simulink model "gm_DVBS_AXI4Stream"  (R2023b)
settings: Solver=FixedStepAuto  StartTime=0.0  StopTime=160000/fs  FixedStep=5e-9  RelTol=1e-3  EnableMultiTasking=on
model workspace (MAT data in the model file):
  HDLVAXIManagerConfig = hdlverifier.internal.AXIMaster.ConfigParams
undefined symbols (not defined in the file or in its folder): ctrlIn, fs, iniStates, n, sourceData
libraries: simulink x12, hdlsllib x9, whdledac x1, commcnvintrlv2 x1, commhdlblkcod x1
settings Model: Creator=31651  LastModifiedBy=31651
settings SolverCC: PositivePriorityOrder=on  AutoInsertRateTranBlk=on
settings DataIOCC: ReturnWorkspaceOutputs=off
settings OptimizationCC: BlockReduction=off  ConditionallyExecuteInputs=off  DefaultParameterBehavior=Inlined  DefaultUnderspecifiedDataType=single  EnhancedBackFolding=on  PassReuseOutputArgsAs=Individual arguments  ZeroExternalMemoryAtStartup=off  ZeroInternalMemoryAtStartup=off  MaxStackSize=64  OptimizeBlockOrder=speed  DifferentSizesBufferReuse=on  OptimizationCustomize=off  EfficientTunableParamExpr=on
settings DebuggingCC: AlgebraicLoopMsg=error  ArtificialAlgebraicLoopMsg=none  InheritedTsInSrcMsg=none  SingleTaskRateTransMsg=error  ParameterPrecisionLossMsg=none  ParameterTunabilityLossMsg=error
settings HardwareCC: ProdBitPerPointer=32  ProdBitPerSizeT=32  ProdBitPerPtrDiffT=32  ProdLargestAtomicFloat=None  ProdIntDivRoundTo=Undefined  ProdEndianess=Unspecified  ProdWordSize=32  ProdHWDeviceType=ASIC/FPGA->ASIC/FPGA  TargetBitPerPointer=64  TargetBitPerSizeT=64  TargetBitPerPtrDiffT=64  TargetLongLongMode=on  TargetIntDivRoundTo=Zero  TargetEndianess=LittleEndian  TargetWordSize=64  TargetHWDeviceType=Custom Processor->MATLAB Host Computer  ProdEqTarget=off  HardwareBoardFeatureSet=SoCBlockset
settings ModelReferenceCC: ModelReferenceNumInstancesAllowed=Single
settings SFSimCC: MATLABDynamicMemAlloc=off
settings RTWCC: Description=Embedded Coder  SystemTargetFile=ert.tlc  TemplateMakefile=ert_default_tmf
settings CodeAppCC: ForceParamTrailComments=on  IgnoreCustomStorageClasses=off  OperatorAnnotations=on  SimulinkDataObjDesc=on  SFDataObjDesc=on  InsertBlockDesc=on
settings ERTTargetCC: ERTCustomFileTemplate=example_file_process.tlc

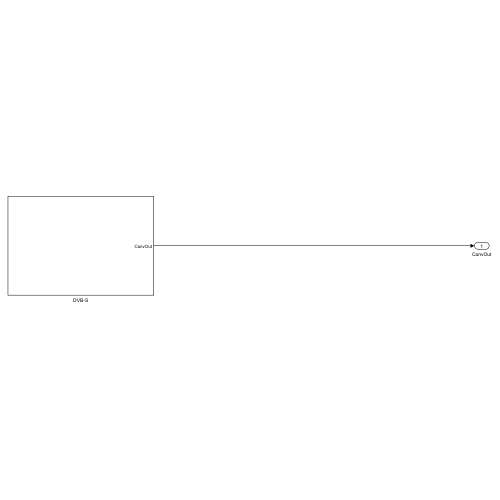
[thumbnail: Simulink's stored preview of the top-level diagram]
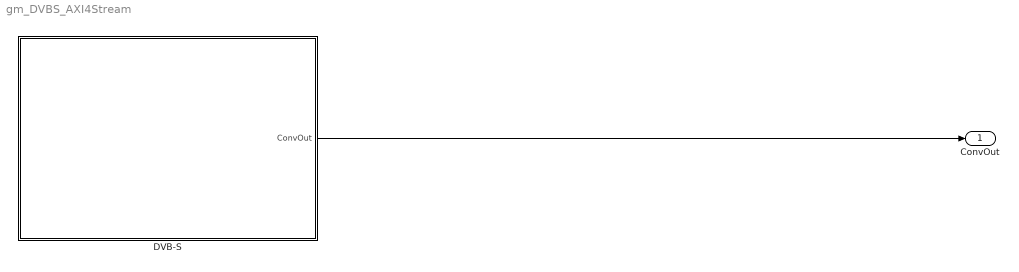
== system gm_DVBS_AXI4Stream ==
  DVB-S : Subsystem
  ConvOut : Outport  VectorParamsAs1DForOutWhenUnconnected=off
  wires:
  DVB-S/1(ConvOut) -> ConvOut/1

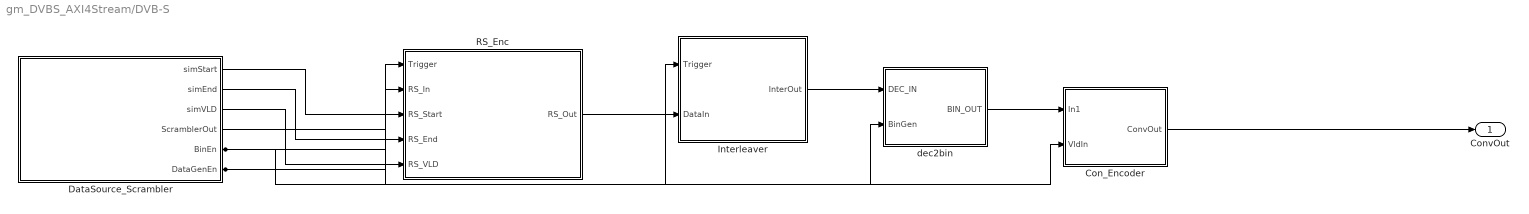
== system gm_DVBS_AXI4Stream/DVB-S ==
  Con_Encoder : Subsystem
  DataSource_Scrambler : Subsystem
  Interleaver : Subsystem
  RS_Enc : Subsystem
  dec2bin : Subsystem
  ConvOut : Outport  SampleTime=5e-09
  wires:
  Con_Encoder/1(ConvOut) -> ConvOut/1
  DataSource_Scrambler/1(simStart) -> RS_Enc/3(RS_Start)
  DataSource_Scrambler/2(simEnd) -> RS_Enc/4(RS_End)
  DataSource_Scrambler/3("simVLD ") -> RS_Enc/5(RS_VLD)
  DataSource_Scrambler/4(ScramblerOut) -> RS_Enc/2(RS_In)
  DataSource_Scrambler/5(BinEn) -> Con_Encoder/2(VldIn), dec2bin/2(BinGen)
  DataSource_Scrambler/6(DataGenEn) -> RS_Enc/1(Trigger), Interleaver/1(Trigger)
  Interleaver/1(InterOut) -> dec2bin/1(DEC_IN)
  RS_Enc/1(RS_Out) -> Interleaver/2(DataIn)
  dec2bin/1(BIN_OUT) -> Con_Encoder/1(In1)

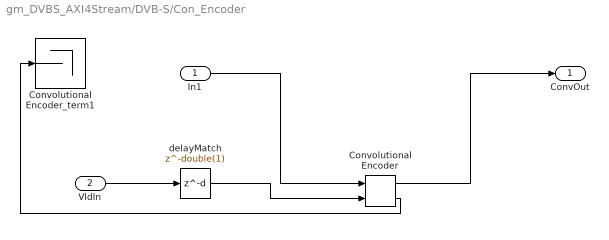
== system gm_DVBS_AXI4Stream/DVB-S/Con_Encoder ==
  In1 : Inport  OutDataTypeStr=boolean  PortDimensions=1  SampleTime=5e-09
  VldIn : Inport  Port=2  OutDataTypeStr=boolean  PortDimensions=1  SampleTime=5e-09
  Convolutional Encoder : whdledac/Convolutional Encoder  ConstraintLength=7  CodeGenerator=[171 133]  FeedbackConnection=0  TerminationMethod=Continuous  ResetPort=off  InitialStatePort=off  FinalStatePort=off  SimulateUsing=Code generation
  Convolutional Encoder_term1 : Terminator
  delayMatch : Delay  DelayLength=double(1)  InitialCondition=0  SampleTime=5e-09
  ConvOut : Outport  SampleTime=5e-09
  wires:
  In1/1 -> Convolutional Encoder/1
  delayMatch/1 -> Convolutional Encoder/2
  Convolutional Encoder/1 -> ConvOut/1
  Convolutional Encoder/2 -> Convolutional Encoder_term1/1
  VldIn/1 -> delayMatch/1

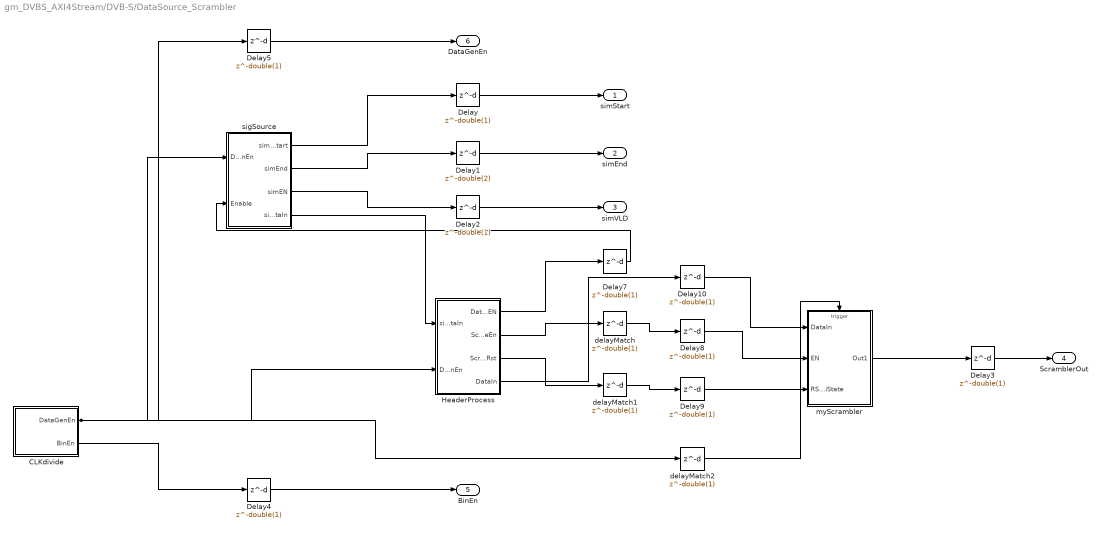
== system gm_DVBS_AXI4Stream/DVB-S/DataSource_Scrambler ==
  CLKdivide : Subsystem
  Delay{,2..5,7..10} (9 alike) : Delay  DelayLength=double(1)  InitialCondition=0  SampleTime=5e-09
  Delay1 : Delay  DelayLength=double(2)  InitialCondition=0  SampleTime=5e-09
  HeaderProcess : Subsystem
  delayMatch : Delay  DelayLength=double(1)  InitialCondition=0  SampleTime=5e-09
  delayMatch1 : Delay  DelayLength=double(1)  InitialCondition=0  SampleTime=5e-09
  delayMatch2 : Delay  DelayLength=double(1)  InitialCondition=0  SampleTime=5e-09
  myScrambler : Subsystem
  sigSource : Subsystem
  simStart : Outport  SampleTime=5e-09
  simEnd : Outport  Port=2  SampleTime=5e-09
  "simVLD " : Outport  Port=3  SampleTime=5e-09
  ScramblerOut : Outport  Port=4  SampleTime=5e-09
  BinEn : Outport  Port=5  SampleTime=5e-09  VectorParamsAs1DForOutWhenUnconnected=off
  DataGenEn : Outport  Port=6  SampleTime=5e-09  VectorParamsAs1DForOutWhenUnconnected=off
  wires:
  delayMatch2/1 -> myScrambler/Trigger
  CLKdivide/2(BinEn) -> Delay4/1
  Delay/1 -> simStart/1
  Delay1/1 -> simEnd/1
  Delay10/1 -> myScrambler/1(DataIn)
  Delay2/1 -> "simVLD "/1
  Delay3/1 -> ScramblerOut/1
  Delay4/1 -> BinEn/1
  Delay5/1 -> DataGenEn/1
  Delay8/1 -> myScrambler/2(EN)
  Delay9/1 -> myScrambler/3(RST_IniState)
  myScrambler/1(Out1) -> Delay3/1
  CLKdivide/1(DataGenEn) -> delayMatch2/1, Delay5/1, sigSource/1(DataGenEn), HeaderProcess/2(DataGenEn)
  delayMatch/1 -> Delay8/1
  delayMatch1/1 -> Delay9/1
  HeaderProcess/1(DataGenEN) -> Delay7/1
  sigSource/1(simStart) -> Delay/1
  sigSource/2(simEnd) -> Delay1/1
  sigSource/3(simEN) -> Delay2/1
  Delay7/1 -> sigSource/2(Enable)
  HeaderProcess/2(ScrambleEn) -> delayMatch/1
  HeaderProcess/3(ScrambleRst) -> delayMatch1/1
  HeaderProcess/4(DataIn) -> Delay10/1
  sigSource/4(simDataIn) -> HeaderProcess/1(simDataIn)

== system gm_DVBS_AXI4Stream/DVB-S/Interleaver ==
  Trigger : Inport  OutDataTypeStr=boolean  PortDimensions=1  SampleTime=5e-09
  DataIn : Inport  Port=2  OutDataTypeStr=uint8  PortDimensions=1  SampleTime=5e-09
  Con_Interleaver : Subsystem
  delayMatch : Delay  DelayLength=double(1)  InitialCondition=0  SampleTime=5e-09
  InterOut : Outport  SampleTime=5e-09
  wires:
  delayMatch/1 -> Con_Interleaver/Trigger
  DataIn/1 -> Con_Interleaver/1(In1)
  Con_Interleaver/1(Out1) -> InterOut/1
  Trigger/1 -> delayMatch/1

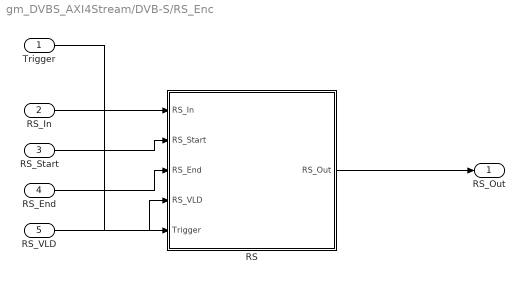
== system gm_DVBS_AXI4Stream/DVB-S/RS_Enc ==
  Trigger : Inport  OutDataTypeStr=boolean  PortDimensions=1  SampleTime=5e-09
  RS_In : Inport  Port=2  OutDataTypeStr=uint8  PortDimensions=1  SampleTime=5e-09
  RS_Start : Inport  Port=3  OutDataTypeStr=boolean  PortDimensions=1  SampleTime=5e-09
  RS_End : Inport  Port=4  OutDataTypeStr=boolean  PortDimensions=1  SampleTime=5e-09
  RS_VLD : Inport  Port=5  OutDataTypeStr=boolean  PortDimensions=1  SampleTime=5e-09
  RS : Subsystem
  RS_Out : Outport  SampleTime=5e-09
  wires:
  Trigger/1 -> RS/5(Trigger)
  RS_In/1 -> RS/1(RS_In)
  RS_Start/1 -> RS/2(RS_Start)
  RS_End/1 -> RS/3(RS_End)
  RS_VLD/1 -> RS/4(RS_VLD)
  RS/1(RS_Out) -> RS_Out/1

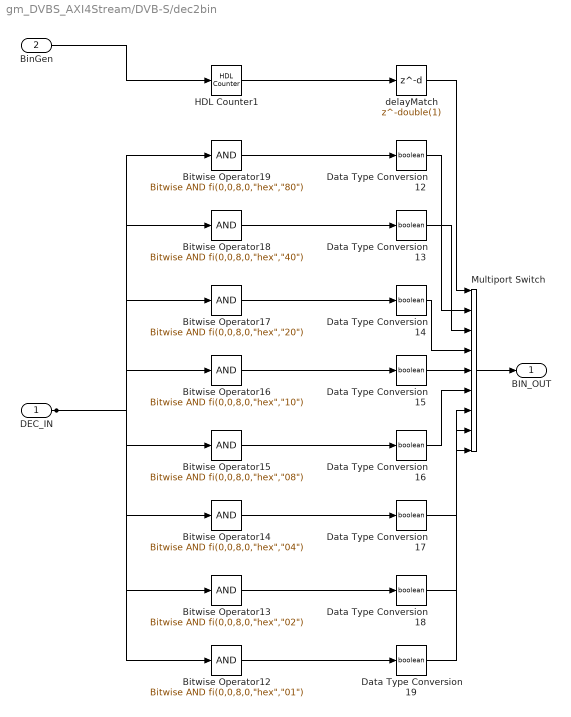
== system gm_DVBS_AXI4Stream/DVB-S/dec2bin ==
  DEC_IN : Inport  OutDataTypeStr=uint8  PortDimensions=1  SampleTime=5e-09
  BinGen : Inport  Port=2  OutDataTypeStr=boolean  PortDimensions=1  SampleTime=5e-09
  Bitwise Operator12 : simulink/Logic and Bit Operations/Bitwise Operator  logicop=AND  UseBitMask=on  BitMask="fi(0,0,8,0,\"hex\",\"01\")"  BitMaskRealWorld=Real World Value
  Bitwise Operator13 : simulink/Logic and Bit Operations/Bitwise Operator  logicop=AND  UseBitMask=on  BitMask="fi(0,0,8,0,\"hex\",\"02\")"  BitMaskRealWorld=Real World Value
  Bitwise Operator14 : simulink/Logic and Bit Operations/Bitwise Operator  logicop=AND  UseBitMask=on  BitMask="fi(0,0,8,0,\"hex\",\"04\")"  BitMaskRealWorld=Real World Value
  Bitwise Operator15 : simulink/Logic and Bit Operations/Bitwise Operator  logicop=AND  UseBitMask=on  BitMask="fi(0,0,8,0,\"hex\",\"08\")"  BitMaskRealWorld=Real World Value
  Bitwise Operator16 : simulink/Logic and Bit Operations/Bitwise Operator  logicop=AND  UseBitMask=on  BitMask="fi(0,0,8,0,\"hex\",\"10\")"  BitMaskRealWorld=Real World Value
  Bitwise Operator17 : simulink/Logic and Bit Operations/Bitwise Operator  logicop=AND  UseBitMask=on  BitMask="fi(0,0,8,0,\"hex\",\"20\")"  BitMaskRealWorld=Real World Value
  Bitwise Operator18 : simulink/Logic and Bit Operations/Bitwise Operator  logicop=AND  UseBitMask=on  BitMask="fi(0,0,8,0,\"hex\",\"40\")"  BitMaskRealWorld=Real World Value
  Bitwise Operator19 : simulink/Logic and Bit Operations/Bitwise Operator  logicop=AND  UseBitMask=on  BitMask="fi(0,0,8,0,\"hex\",\"80\")"  BitMaskRealWorld=Real World Value
  Data Type Conversion{12..19} (8 alike) : DataTypeConversion  OutDataTypeStr=boolean  SampleTime=5e-09  SaturateOnIntegerOverflow=off  RndMeth=Floor
  HDL Counter1 : hdlsllib/Sources/HDL Counter  CountType=Count limited  CountInit=1  CountStep=1  CountMax=8  CountFromType=Specify  CountFrom=1  CountResetPort=off  CountLoadPort=off  CountEnbPort=on  CountDirPort=off  CountHitOutputPort=off  CountDataType=Unsigned  CountWordLen=8  CountFracLen=0  CountSampTime=1/fs
  Multiport Switch : MultiPortSwitch  Inputs=8  DiagnosticForDefault=None  SampleTime=5e-09  SaturateOnIntegerOverflow=off  InputSameDT=off
  delayMatch : Delay  DelayLength=double(1)  InitialCondition=0  SampleTime=5e-09
  BIN_OUT : Outport  SampleTime=5e-09
  wires:
  DEC_IN/1 -> Bitwise Operator19/1, Bitwise Operator18/1, Bitwise Operator17/1, Bitwise Operator16/1, Bitwise Operator15/1, Bitwise Operator14/1, Bitwise Operator13/1, Bitwise Operator12/1
  BinGen/1 -> HDL Counter1/1
  Bitwise Operator12/1 -> Data Type Conversion19/1
  Bitwise Operator13/1 -> Data Type Conversion18/1
  Bitwise Operator14/1 -> Data Type Conversion17/1
  Bitwise Operator15/1 -> Data Type Conversion16/1
  Bitwise Operator16/1 -> Data Type Conversion15/1
  Bitwise Operator17/1 -> Data Type Conversion14/1
  Bitwise Operator18/1 -> Data Type Conversion13/1
  Bitwise Operator19/1 -> Data Type Conversion12/1
  Data Type Conversion12/1 -> Multiport Switch/2
  Data Type Conversion13/1 -> Multiport Switch/3
  Data Type Conversion14/1 -> Multiport Switch/4
  Data Type Conversion15/1 -> Multiport Switch/5
  Data Type Conversion16/1 -> Multiport Switch/6
  Data Type Conversion17/1 -> Multiport Switch/7
  Data Type Conversion18/1 -> Multiport Switch/8
  Data Type Conversion19/1 -> Multiport Switch/9
  delayMatch/1 -> Multiport Switch/1
  Multiport Switch/1 -> BIN_OUT/1
  HDL Counter1/1 -> delayMatch/1

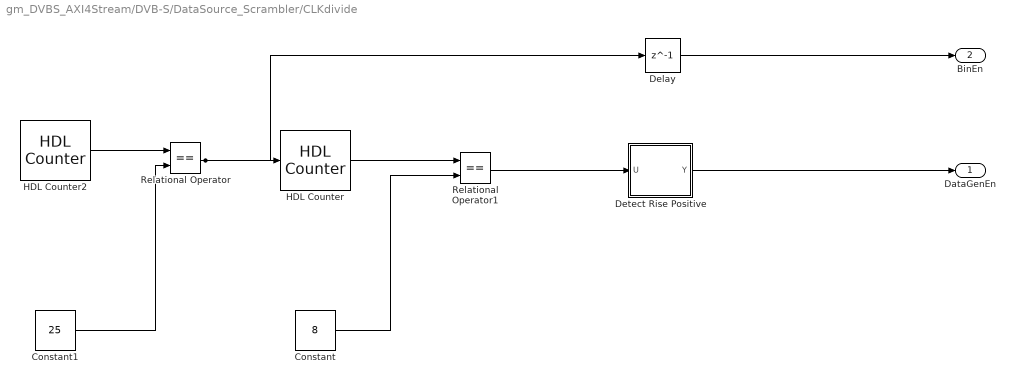
== system gm_DVBS_AXI4Stream/DVB-S/DataSource_Scrambler/CLKdivide ==
  Constant : Constant  Value=8  VectorParams1D=off  OutDataTypeStr=uint8  SampleTime=1/fs
  Constant1 : Constant  Value=25  VectorParams1D=off  OutDataTypeStr=uint8  SampleTime=1/fs
  Delay : Delay  DelayLength=1
  Detect Rise Positive : Subsystem  mask(Detect Rise Positive){vinit=double(0), InputProcessing=Elements as channels (sample based), OutDataTypeStr=boolean}
      mask prompts: vinit "Simulink:masks:InitialCondition_MP"; InputProcessing "Simulink:masks:InputProcessing_MP"; OutDataTypeStr "Simulink:masks:OutputDataType_MP"
      mask help: Simulink:masks:DetectRisePositive_MD
      mask init:
      | InputProcessing = 'Elements as channels (sample based)';
      | OutDataTypeStr = 'boolean';
      | vinit = double(0);
      mask TypeOptions InputProcessing: Simulink:masks:ColumnsAsChannelsFrameBased | Simulink:masks:ElementsAsChannelsSampleBased
      mask TypeOptions OutDataTypeStr: Simulink:masks:uint8 | Simulink:masks:boolean
      mask Display: fprintf('U > 0\n&  NOT\nU/z > 0')
  HDL Counter : hdlsllib/Sources/HDL Counter  CountType=Count limited  CountInit=1  CountStep=1  CountMax=8  CountFromType=Initial value  CountFrom=1  CountResetPort=off  CountLoadPort=off  CountEnbPort=on  CountDirPort=off  CountHitOutputPort=off  CountDataType=Unsigned  CountWordLen=8  CountFracLen=0  CountSampTime=1
  HDL Counter2 : hdlsllib/Sources/HDL Counter  CountType=Count limited  CountInit=1  CountStep=1  CountMax=25  CountFromType=Initial value  CountFrom=1  CountResetPort=off  CountLoadPort=off  CountEnbPort=off  CountDirPort=off  CountHitOutputPort=off  CountDataType=Unsigned  CountWordLen=8  CountFracLen=0  CountSampTime=1/fs
  Relational Operator : RelationalOperator  Operator===  OutDataTypeStr=boolean  InputSameDT=off
  Relational Operator1 : RelationalOperator  Operator===  OutDataTypeStr=boolean  InputSameDT=off
  DataGenEn : Outport  SampleTime=5e-09  VectorParamsAs1DForOutWhenUnconnected=off
  BinEn : Outport  Port=2  SampleTime=5e-09  VectorParamsAs1DForOutWhenUnconnected=off
  wires:
  Constant/1 -> Relational Operator1/2
  Constant1/1 -> Relational Operator/2
  Delay/1 -> BinEn/1
  Detect Rise Positive/1(Y) -> DataGenEn/1
  HDL Counter/1 -> Relational Operator1/1
  HDL Counter2/1 -> Relational Operator/1
  Relational Operator/1 -> Delay/1, HDL Counter/1
  Relational Operator1/1 -> Detect Rise Positive/1(U)

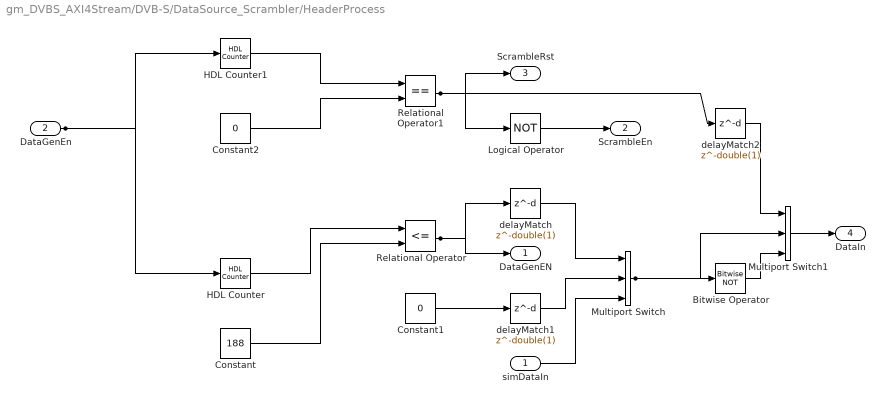
== system gm_DVBS_AXI4Stream/DVB-S/DataSource_Scrambler/HeaderProcess ==
  simDataIn : Inport  OutDataTypeStr=uint8  PortDimensions=1  SampleTime=5e-09
  DataGenEn : Inport  Port=2  OutDataTypeStr=boolean  PortDimensions=1  SampleTime=5e-09
  Bitwise Operator : simulink/Logic and Bit Operations/Bitwise Operator  logicop=NOT  UseBitMask=off  BitMask=double(0)  BitMaskRealWorld=Real World Value
  Constant : Constant  Value=188  OutDataTypeStr=uint8  SampleTime=5e-09
  Constant1 : Constant  Value=0  OutDataTypeStr=uint8  SampleTime=5e-09
  Constant2 : Constant  Value=0  OutDataTypeStr=uint8  SampleTime=5e-09
  HDL Counter : hdlsllib/Sources/HDL Counter  CountType=Count limited  CountInit=1  CountStep=1  CountMax=n  CountFromType=Initial value  CountFrom=1  CountResetPort=off  CountLoadPort=off  CountEnbPort=on  CountDirPort=off  CountHitOutputPort=off  CountDataType=Unsigned  CountWordLen=8  CountFracLen=0  CountSampTime=1/fs
  HDL Counter1 : hdlsllib/Sources/HDL Counter  CountType=Count limited  CountInit=0  CountStep=1  CountMax=n*8-1  CountFromType=Initial value  CountFrom=0  CountResetPort=off  CountLoadPort=off  CountEnbPort=on  CountDirPort=off  CountHitOutputPort=off  CountDataType=Unsigned  CountWordLen=16  CountFracLen=0  CountSampTime=1/fs
  Logical Operator : Logic  Operator=NOT  Inputs=1  AllPortsSameDT=off  OutDataTypeStr=boolean  SampleTime=5e-09
  Multiport Switch : MultiPortSwitch  DataPortOrder=Specify indices  Inputs=2  DataPortIndices={ double(0) double(1)}  DiagnosticForDefault=None  OutDataTypeStr=uint8  SampleTime=5e-09  SaturateOnIntegerOverflow=off  InputSameDT=off
  Multiport Switch1 : MultiPortSwitch  DataPortOrder=Specify indices  Inputs=2  DataPortIndices={ double(0) double(1)}  DiagnosticForDefault=None  OutDataTypeStr=uint8  SampleTime=5e-09  SaturateOnIntegerOverflow=off  InputSameDT=off
  Relational Operator : RelationalOperator  Operator=<=  OutDataTypeStr=boolean  SampleTime=5e-09  InputSameDT=off
  Relational Operator1 : RelationalOperator  Operator===  OutDataTypeStr=boolean  SampleTime=5e-09  InputSameDT=off
  delayMatch : Delay  DelayLength=double(1)  InitialCondition=0  SampleTime=5e-09
  delayMatch1 : Delay  DelayLength=double(1)  InitialCondition=0  SampleTime=5e-09
  delayMatch2 : Delay  DelayLength=double(1)  InitialCondition=0  SampleTime=5e-09
  DataGenEN : Outport  SampleTime=5e-09  VectorParamsAs1DForOutWhenUnconnected=off
  ScrambleEn : Outport  Port=2  SampleTime=5e-09  VectorParamsAs1DForOutWhenUnconnected=off
  ScrambleRst : Outport  Port=3  SampleTime=5e-09  VectorParamsAs1DForOutWhenUnconnected=off
  DataIn : Outport  Port=4  SampleTime=5e-09
  wires:
  simDataIn/1 -> Multiport Switch/3
  DataGenEn/1 -> HDL Counter/1, HDL Counter1/1
  Bitwise Operator/1 -> Multiport Switch1/3
  Constant/1 -> Relational Operator/2
  delayMatch1/1 -> Multiport Switch/2
  Constant2/1 -> Relational Operator1/2
  HDL Counter/1 -> Relational Operator/1
  HDL Counter1/1 -> Relational Operator1/1
  Logical Operator/1 -> ScrambleEn/1
  Multiport Switch/1 -> Multiport Switch1/2, Bitwise Operator/1
  Multiport Switch1/1 -> DataIn/1
  delayMatch/1 -> Multiport Switch/1
  delayMatch2/1 -> Multiport Switch1/1
  Relational Operator/1 -> delayMatch/1, DataGenEN/1
  Constant1/1 -> delayMatch1/1
  Relational Operator1/1 -> delayMatch2/1, Logical Operator/1, ScrambleRst/1

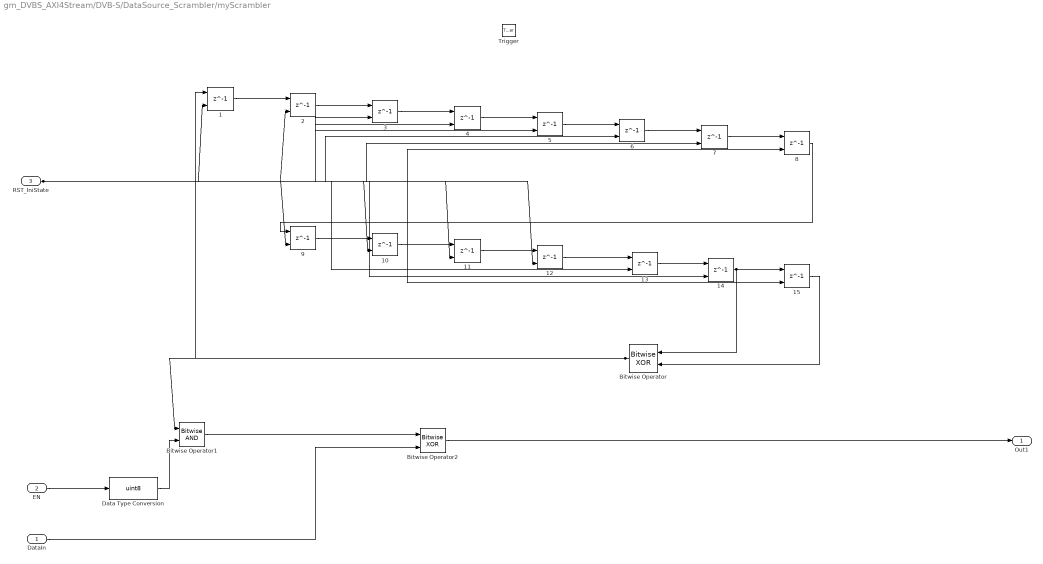
== system gm_DVBS_AXI4Stream/DVB-S/DataSource_Scrambler/myScrambler ==
  DataIn : Inport  OutDataTypeStr=uint8  PortDimensions=1
  EN : Inport  Port=2  OutDataTypeStr=boolean  PortDimensions=1
  RST_IniState : Inport  Port=3  OutDataTypeStr=boolean  PortDimensions=1
  Trigger : TriggerPort  VariantControl=(inherit)  PortDimensions=1  OutDataTypeStr=boolean
  1 : Delay  DelayLength=1  InitialCondition=iniStates(1)  ExternalReset=Level
      settings: InputPortMap=u0,r5
  10 : Delay  DelayLength=1  InitialCondition=iniStates(10)  ExternalReset=Level
      settings: InputPortMap=u0,r5
  11 : Delay  DelayLength=1  InitialCondition=iniStates(11)  ExternalReset=Level
      settings: InputPortMap=u0,r5
  12 : Delay  DelayLength=1  InitialCondition=iniStates(12)  ExternalReset=Level
      settings: InputPortMap=u0,r5
  13 : Delay  DelayLength=1  InitialCondition=iniStates(13)  ExternalReset=Level
      settings: InputPortMap=u0,r5
  14 : Delay  DelayLength=1  InitialCondition=iniStates(14)  ExternalReset=Level
      settings: InputPortMap=u0,r5
  15 : Delay  DelayLength=1  InitialCondition=iniStates(15)  ExternalReset=Level
      settings: InputPortMap=u0,r5
  2 : Delay  DelayLength=1  InitialCondition=iniStates(2)  ExternalReset=Level
      settings: InputPortMap=u0,r5
  3 : Delay  DelayLength=1  InitialCondition=iniStates(3)  ExternalReset=Level
      settings: InputPortMap=u0,r5
  4 : Delay  DelayLength=1  InitialCondition=iniStates(4)  ExternalReset=Level
      settings: InputPortMap=u0,r5
  5 : Delay  DelayLength=1  InitialCondition=iniStates(5)  ExternalReset=Level
      settings: InputPortMap=u0,r5
  6 : Delay  DelayLength=1  InitialCondition=iniStates(6)  ExternalReset=Level
      settings: InputPortMap=u0,r5
  7 : Delay  DelayLength=1  InitialCondition=iniStates(7)  ExternalReset=Level
      settings: InputPortMap=u0,r5
  8 : Delay  DelayLength=1  InitialCondition=iniStates(8)  ExternalReset=Level
      settings: InputPortMap=u0,r5
  9 : Delay  DelayLength=1  InitialCondition=iniStates(9)  ExternalReset=Level
      settings: InputPortMap=u0,r5
  Bitwise Operator : simulink/Logic and Bit Operations/Bitwise Operator  logicop=XOR  UseBitMask=off  NumInputPorts=2  BitMask=bin2dec('11011001')  BitMaskRealWorld=Stored Integer
  Bitwise Operator1 : simulink/Logic and Bit Operations/Bitwise Operator  logicop=AND  UseBitMask=off  NumInputPorts=2  BitMask=bin2dec('11011001')  BitMaskRealWorld=Stored Integer
  Bitwise Operator2 : simulink/Logic and Bit Operations/Bitwise Operator  logicop=XOR  UseBitMask=off  NumInputPorts=2  BitMask=bin2dec('11011001')  BitMaskRealWorld=Stored Integer
  Data Type Conversion : DataTypeConversion  OutDataTypeStr=uint8  SaturateOnIntegerOverflow=off  RndMeth=Floor
  Out1 : Outport  InitialOutput=0
  wires:
  DataIn/1 -> Bitwise Operator2/2
  EN/1 -> Data Type Conversion/1
  RST_IniState/1 -> 14/2, 13/2, 12/2, 11/2, 10/2, 9/2, 8/2, 7/2, 6/2, 5/2, 4/2, 3/2, 2/2, 1/2, 15/2
  Bitwise Operator/1 -> Bitwise Operator1/1, 1/1
  Bitwise Operator1/1 -> Bitwise Operator2/1
  Bitwise Operator2/1 -> Out1/1
  Data Type Conversion/1 -> Bitwise Operator1/2
  15/1 -> Bitwise Operator/2
  1/1 -> 2/1
  2/1 -> 3/1
  3/1 -> 4/1
  4/1 -> 5/1
  5/1 -> 6/1
  6/1 -> 7/1
  7/1 -> 8/1
  8/1 -> 9/1
  9/1 -> 10/1
  10/1 -> 11/1
  11/1 -> 12/1
  12/1 -> 13/1
  13/1 -> 14/1
  14/1 -> Bitwise Operator/1, 15/1

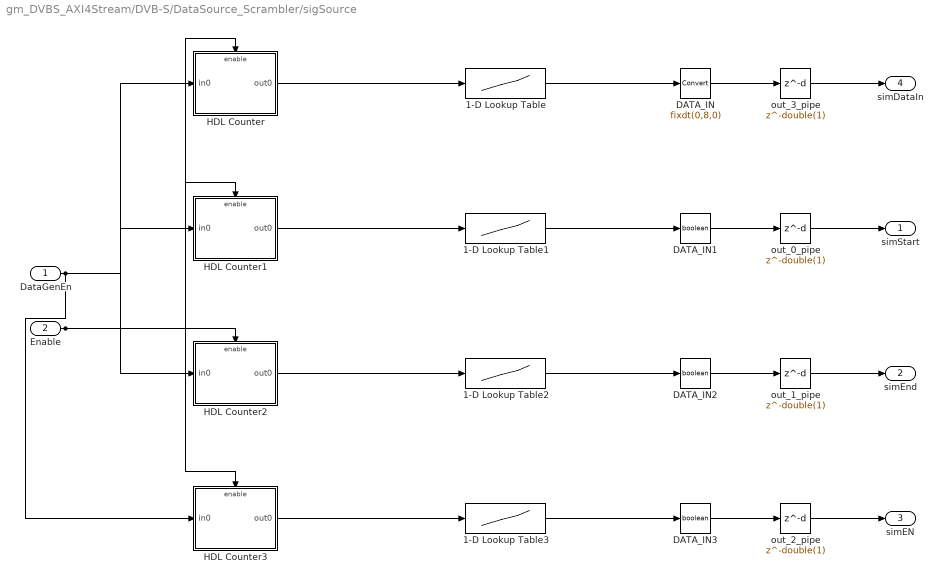
== system gm_DVBS_AXI4Stream/DVB-S/DataSource_Scrambler/sigSource ==
  DataGenEn : Inport  OutDataTypeStr=boolean  PortDimensions=1  SampleTime=5e-09
  Enable : Inport  Port=2  OutDataTypeStr=boolean  SampleTime=5e-09
  1-D Lookup Table : Lookup_n-D  NumberOfTableDimensions=1  LookupTableObject=''  BreakpointsForDimension1=[0:18800-1]'  BreakpointsForDimension1FirstPoint=10  BreakpointsForDimension2FirstPoint=10  BreakpointsForDimension1Spacing=12  BreakpointsForDimension2Spacing=12  IndexSearchMethod=Evenly spaced points  Table=sourceData  InterpMethod=Flat  InternalRulePriority=Speed  OutDataTypeStr=uint8  RndMeth=Simplest
  1-D Lookup Table1 : Lookup_n-D  NumberOfTableDimensions=1  LookupTableObject=''  BreakpointsForDimension1=[0:204-1]'  BreakpointsForDimension1FirstPoint=10  BreakpointsForDimension2FirstPoint=10  BreakpointsForDimension1Spacing=12  BreakpointsForDimension2Spacing=12  IndexSearchMethod=Evenly spaced points  Table=ctrlIn(:,1)  InterpMethod=Flat  InternalRulePriority=Speed  OutDataTypeStr=uint8  RndMeth=Simplest
  1-D Lookup Table2 : Lookup_n-D  NumberOfTableDimensions=1  LookupTableObject=''  BreakpointsForDimension1=[0:204-1]'  BreakpointsForDimension1FirstPoint=10  BreakpointsForDimension2FirstPoint=10  BreakpointsForDimension1Spacing=12  BreakpointsForDimension2Spacing=12  IndexSearchMethod=Evenly spaced points  Table=ctrlIn(:,2)  InterpMethod=Flat  InternalRulePriority=Speed  OutDataTypeStr=uint8  RndMeth=Simplest
  1-D Lookup Table3 : Lookup_n-D  NumberOfTableDimensions=1  LookupTableObject=''  BreakpointsForDimension1=[0:204-1]'  BreakpointsForDimension1FirstPoint=10  BreakpointsForDimension2FirstPoint=10  BreakpointsForDimension1Spacing=12  BreakpointsForDimension2Spacing=12  IndexSearchMethod=Evenly spaced points  Table=ctrlIn(:,3)  InterpMethod=Flat  InternalRulePriority=Speed  OutDataTypeStr=uint8  RndMeth=Simplest
  DATA_IN : DataTypeConversion  OutDataTypeStr=fixdt(0,8,0)
  DATA_IN1 : DataTypeConversion  OutDataTypeStr=boolean  SampleTime=5e-09  SaturateOnIntegerOverflow=off  RndMeth=Floor
  DATA_IN2 : DataTypeConversion  OutDataTypeStr=boolean  SampleTime=5e-09  SaturateOnIntegerOverflow=off  RndMeth=Floor
  DATA_IN3 : DataTypeConversion  OutDataTypeStr=boolean  SampleTime=5e-09  SaturateOnIntegerOverflow=off  RndMeth=Floor
  HDL Counter : Subsystem
      settings: MinAlgLoopOccurrences=on
  HDL Counter1 : Subsystem
      settings: MinAlgLoopOccurrences=on
  HDL Counter2 : Subsystem
      settings: MinAlgLoopOccurrences=on
  HDL Counter3 : Subsystem
      settings: MinAlgLoopOccurrences=on
  out_0_pipe : Delay  DelayLength=double(1)  InitialCondition=0
  out_1_pipe : Delay  DelayLength=double(1)  InitialCondition=0
  out_2_pipe : Delay  DelayLength=double(1)  InitialCondition=0
  out_3_pipe : Delay  DelayLength=double(1)  InitialCondition=0
  simStart : Outport  SampleTime=5e-09  InitialOutput=0
  simEnd : Outport  Port=2  SampleTime=5e-09  InitialOutput=0
  simEN : Outport  Port=3  SampleTime=5e-09  InitialOutput=0
  simDataIn : Outport  Port=4  SampleTime=5e-09  InitialOutput=0
  wires:
  Enable/1 -> HDL Counter3/Enable, HDL Counter2/Enable, HDL Counter1/Enable, HDL Counter/Enable
  DataGenEn/1 -> HDL Counter3/1(in0), HDL Counter2/1(in0), HDL Counter1/1(in0), HDL Counter/1(in0)
  1-D Lookup Table/1 -> DATA_IN/1
  1-D Lookup Table1/1 -> DATA_IN1/1
  1-D Lookup Table2/1 -> DATA_IN2/1
  1-D Lookup Table3/1 -> DATA_IN3/1
  DATA_IN/1 -> out_3_pipe/1
  DATA_IN1/1 -> out_0_pipe/1
  DATA_IN2/1 -> out_1_pipe/1
  DATA_IN3/1 -> out_2_pipe/1
  HDL Counter/1(out0) -> 1-D Lookup Table/1
  HDL Counter1/1(out0) -> 1-D Lookup Table1/1
  HDL Counter2/1(out0) -> 1-D Lookup Table2/1
  HDL Counter3/1(out0) -> 1-D Lookup Table3/1
  out_0_pipe/1 -> simStart/1
  out_1_pipe/1 -> simEnd/1
  out_2_pipe/1 -> simEN/1
  out_3_pipe/1 -> simDataIn/1

== system gm_DVBS_AXI4Stream/DVB-S/Interleaver/Con_Interleaver ==
  In1 : Inport  OutDataTypeStr=uint8  PortDimensions=1
  Trigger : TriggerPort  VariantControl=(inherit)  PortDimensions=1  OutDataTypeStr=boolean
  Convolutional Interleaver : commcnvintrlv2/Convolutional Interleaver  N=12  B=17  ic=0
      settings: LibrarySourceBlock=|
      | commhdlinterleave/Convolutional
      | Interleaver
  Out1 : Outport  InitialOutput=0
  wires:
  In1/1 -> Convolutional Interleaver/1
  Convolutional Interleaver/1 -> Out1/1

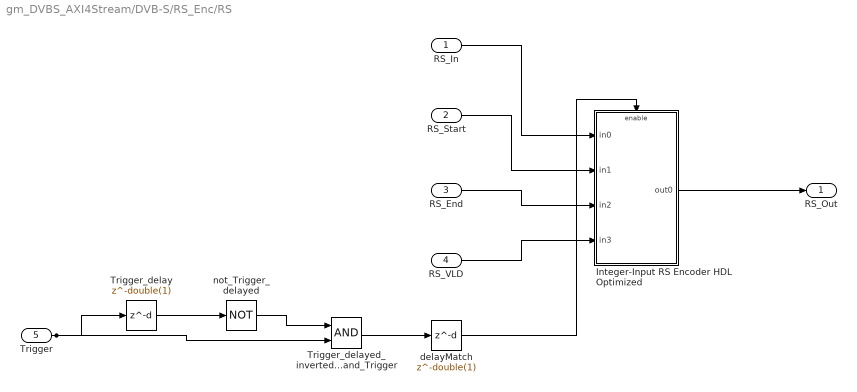
== system gm_DVBS_AXI4Stream/DVB-S/RS_Enc/RS ==
  RS_In : Inport  OutDataTypeStr=uint8  PortDimensions=1  SampleTime=5e-09
  RS_Start : Inport  Port=2  OutDataTypeStr=boolean  PortDimensions=1  SampleTime=5e-09
  RS_End : Inport  Port=3  OutDataTypeStr=boolean  PortDimensions=1  SampleTime=5e-09
  RS_VLD : Inport  Port=4  OutDataTypeStr=boolean  PortDimensions=1  SampleTime=5e-09
  Trigger : Inport  Port=5  OutDataTypeStr=boolean  SampleTime=5e-09
  Integer-Input RS Encoder HDL Optimized : Subsystem
      settings: MinAlgLoopOccurrences=on
  Trigger_delay : Delay  DelayLength=double(1)  InitialCondition=1
  Trigger_delayed_inverted_and_Trigger : Logic  AllPortsSameDT=off  OutDataTypeStr=boolean  SampleTime=5e-09
  delayMatch : Delay  DelayLength=double(1)  InitialCondition=0
  not_Trigger_delayed : Logic  Operator=NOT  Inputs=1  AllPortsSameDT=off  OutDataTypeStr=boolean  SampleTime=5e-09
  RS_Out : Outport  OutDataTypeStr=uint8  SampleTime=5e-09  InitialOutput=0
  wires:
  Trigger/1 -> Trigger_delayed_inverted_and_Trigger/2, Trigger_delay/1
  RS_In/1 -> Integer-Input RS Encoder HDL Optimized/1(in0)
  RS_Start/1 -> Integer-Input RS Encoder HDL Optimized/2(in1)
  RS_End/1 -> Integer-Input RS Encoder HDL Optimized/3(in2)
  RS_VLD/1 -> Integer-Input RS Encoder HDL Optimized/4(in3)
  Integer-Input RS Encoder HDL Optimized/1(out0) -> RS_Out/1
  Trigger_delay/1 -> not_Trigger_delayed/1
  not_Trigger_delayed/1 -> Trigger_delayed_inverted_and_Trigger/1
  delayMatch/1 -> Integer-Input RS Encoder HDL Optimized/Enable
  Trigger_delayed_inverted_and_Trigger/1 -> delayMatch/1

== system gm_DVBS_AXI4Stream/DVB-S/DataSource_Scrambler/CLKdivide/Detect Rise Positive ==
  note: Edge
  note: U(k)
  U : Inport  OutDataTypeStr=boolean  SampleTime=5e-09
  Delay Input1 : UnitDelay  Description=Store in Global RAM  DisableCoverage=on  InitialCondition=vinit  SampleTime=-1  HasFrameUpgradeWarning=on
  FixPt Relational Operator : RelationalOperator  Operator=>  OutDataTypeStr=boolean  ZeroCross=off  InputSameDT=off
  Positive : Subsystem  mask(Compare To Zero){relop=>, OutDataTypeStr=boolean, ZeroCross=off}
      mask prompts: relop "Simulink:masks:Operator_MP"; OutDataTypeStr "Simulink:masks:OutputDataType_MP"; ZeroCross "Simulink:masks:EnableZerocrossingDetection_MP"
      mask help: Simulink:masks:CompareToZero_MD
      mask init:
      | OutDataTypeStr = 'boolean';
      | ZeroCross = 'off';
      | blkName = 'DVBS_AXI4Stream/DVB-S/DataSource_Scrambler/CLKdivide/Detect Rise\nPositive/Positive';
      | relop = '>';
      | setValue = 'boolean';
      mask TypeOptions relop: == | ~= | < | <= | >= | >
      mask TypeOptions OutDataTypeStr: Simulink:masks:uint8 | Simulink:masks:boolean
      mask Callback ZeroCross: sl('zeroCrossEnable', gcbh);
      mask Display: disp([relop,' 0'])
  Y : Outport  SampleTime=5e-09
  wires:
  U/1 -> Positive/1(u)
  Delay Input1/1 -> FixPt Relational Operator/2
  FixPt Relational Operator/1 -> Y/1
  Positive/1(y) -> FixPt Relational Operator/1, Delay Input1/1

== system gm_DVBS_AXI4Stream/DVB-S/DataSource_Scrambler/sigSource/HDL Counter ==
  in0 : Inport  OutDataTypeStr=boolean  SampleTime=5e-09
  Enable_out2 : EnablePort  OutDataTypeStr=boolean
  HDL Counter : hdlsllib/Sources/HDL Counter  CountType=Count limited  CountInit=0  CountStep=1  CountMax=18800-1  CountFromType=Initial value  CountFrom=0  CountResetPort=off  CountLoadPort=off  CountEnbPort=on  CountDirPort=off  CountHitOutputPort=off  CountDataType=Unsigned  CountWordLen=32  CountFracLen=0  CountSampTime=1/fs
  out0 : Outport  OutDataTypeStr=uint32  SampleTime=5e-09  InitialOutput=0
  wires:
  HDL Counter/1 -> out0/1
  in0/1 -> HDL Counter/1

== system gm_DVBS_AXI4Stream/DVB-S/DataSource_Scrambler/sigSource/HDL Counter1 ==
  in0 : Inport  OutDataTypeStr=boolean  SampleTime=5e-09
  Enable_out2 : EnablePort  OutDataTypeStr=boolean
  HDL Counter1 : hdlsllib/Sources/HDL Counter  CountType=Count limited  CountInit=0  CountStep=1  CountMax=204-1  CountFromType=Initial value  CountFrom=0  CountResetPort=off  CountLoadPort=off  CountEnbPort=on  CountDirPort=off  CountHitOutputPort=off  CountDataType=Unsigned  CountWordLen=8  CountFracLen=0  CountSampTime=1/fs
  out0 : Outport  OutDataTypeStr=uint8  SampleTime=5e-09  InitialOutput=0
  wires:
  HDL Counter1/1 -> out0/1
  in0/1 -> HDL Counter1/1

== system gm_DVBS_AXI4Stream/DVB-S/DataSource_Scrambler/sigSource/HDL Counter2 ==
  in0 : Inport  OutDataTypeStr=boolean  SampleTime=5e-09
  Enable_out2 : EnablePort  OutDataTypeStr=boolean
  HDL Counter2 : hdlsllib/Sources/HDL Counter  CountType=Count limited  CountInit=0  CountStep=1  CountMax=204-1  CountFromType=Initial value  CountFrom=0  CountResetPort=off  CountLoadPort=off  CountEnbPort=on  CountDirPort=off  CountHitOutputPort=off  CountDataType=Unsigned  CountWordLen=8  CountFracLen=0  CountSampTime=1/fs
  out0 : Outport  OutDataTypeStr=uint8  SampleTime=5e-09  InitialOutput=0
  wires:
  HDL Counter2/1 -> out0/1
  in0/1 -> HDL Counter2/1

== system gm_DVBS_AXI4Stream/DVB-S/DataSource_Scrambler/sigSource/HDL Counter3 ==
  in0 : Inport  OutDataTypeStr=boolean  SampleTime=5e-09
  Enable_out2 : EnablePort  OutDataTypeStr=boolean
  HDL Counter3 : hdlsllib/Sources/HDL Counter  CountType=Count limited  CountInit=0  CountStep=1  CountMax=204-1  CountFromType=Initial value  CountFrom=0  CountResetPort=off  CountLoadPort=off  CountEnbPort=on  CountDirPort=off  CountHitOutputPort=off  CountDataType=Unsigned  CountWordLen=8  CountFracLen=0  CountSampTime=1/fs
  out0 : Outport  OutDataTypeStr=uint8  SampleTime=5e-09  InitialOutput=0
  wires:
  HDL Counter3/1 -> out0/1
  in0/1 -> HDL Counter3/1

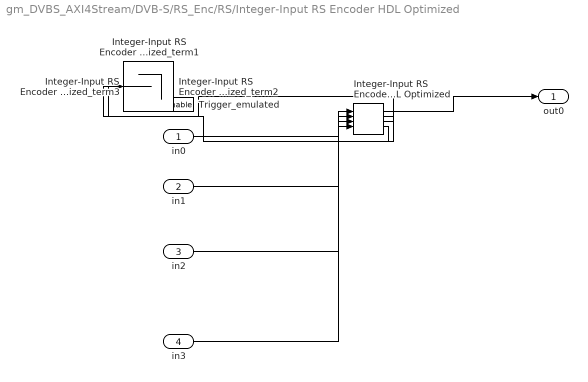
== system gm_DVBS_AXI4Stream/DVB-S/RS_Enc/RS/Integer-Input RS Encoder HDL Optimized ==
  in0 : Inport  OutDataTypeStr=uint8  SampleTime=5e-09
  in1 : Inport  Port=2  OutDataTypeStr=boolean  SampleTime=5e-09
  in2 : Inport  Port=3  OutDataTypeStr=boolean  SampleTime=5e-09
  in3 : Inport  Port=4  OutDataTypeStr=boolean  SampleTime=5e-09
  Trigger_emulated : EnablePort  OutDataTypeStr=boolean
  Integer-Input RS Encoder HDL Optimized : commhdlblkcod/Integer-Input RS Encoder HDL Optimized  CodewordLength=n  MessageLength=k  PrimitivePolynomialSource=Property  PrimitivePolynomial=[1 0 0 0 1 1 1 0 1]  PuncturePatternSource=None  PuncturePattern=[ ones( 2, 1 ); zeros( 2, 1 ) ]  BSource=Property  B=0  SimulateUsing=Code generation
  Integer-Input RS Encoder HDL Optimized_term1 : Terminator
  Integer-Input RS Encoder HDL Optimized_term2 : Terminator
  Integer-Input RS Encoder HDL Optimized_term3 : Terminator
  out0 : Outport  OutDataTypeStr=uint8  SampleTime=5e-09  InitialOutput=0
  wires:
  Integer-Input RS Encoder HDL Optimized/1 -> out0/1
  Integer-Input RS Encoder HDL Optimized/2 -> Integer-Input RS Encoder HDL Optimized_term1/1
  Integer-Input RS Encoder HDL Optimized/3 -> Integer-Input RS Encoder HDL Optimized_term2/1
  Integer-Input RS Encoder HDL Optimized/4 -> Integer-Input RS Encoder HDL Optimized_term3/1
  in0/1 -> Integer-Input RS Encoder HDL Optimized/1
  in1/1 -> Integer-Input RS Encoder HDL Optimized/2
  in2/1 -> Integer-Input RS Encoder HDL Optimized/3
  in3/1 -> Integer-Input RS Encoder HDL Optimized/4

== system gm_DVBS_AXI4Stream/DVB-S/DataSource_Scrambler/CLKdivide/Detect Rise Positive/Positive ==
  u : Inport  OutDataTypeStr=boolean  SampleTime=5e-09
  Compare : RelationalOperator  Operator=>  OutDataTypeStr=boolean  ZeroCross=off
  Constant : Constant  DisableCoverage=on  Value=0  OutDataTypeStr=Inherit: Inherit via back propagation  SampleTime=-1  PreserveConstantTs=on
  y : Outport  SampleTime=5e-09
  wires:
  u/1 -> Compare/1
  Compare/1 -> y/1
  Constant/1 -> Compare/2
